simulink model "modelo_lqr_infinito"  (R2016a)
settings: Solver=VariableStepAuto  StartTime=0.0  StopTime=100  RelTol=1e-3
values from neighbouring files (symbols this model uses):
  A = [-0.1107 0; 0.1107 -0.1107]    [plantilla_lqr.m]
  B = [-1 1;0 0]    [plantilla_lqr.m]
undefined symbols (not defined in the file or in its folder): K
settings Model: Creator=Juan Pablo Requez  LastModifiedBy=Juan Pablo Requez

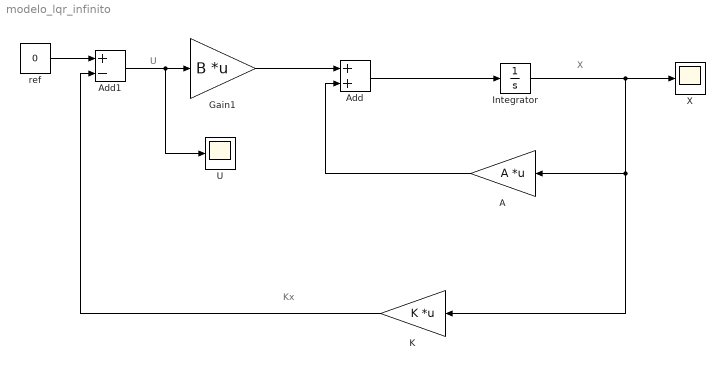
== system modelo_lqr_infinito ==
  note: Kx
  note: U
  note: X
  A : Gain  Gain=A  Multiplication=Matrix(K*u)
  Add : Sum
  Add1 : Sum  Inputs=+-
  Gain1 : Gain  Gain=B  Multiplication=Matrix(K*u)
  Integrator : Integrator  InitialCondition=[0.1 0.1]
  K : Gain  Gain=K  Multiplication=Matrix(K*u)
  U : Scope
  X : Scope
  ref : Constant  Value=0
  wires:
  Integrator/1 -> K/1, A/1, X/1
  A/1 -> Add/2
  Gain1/1 -> Add/1
  Add/1 -> Integrator/1
  Add1/1 -> U/1, Gain1/1
  ref/1 -> Add1/1
  K/1 -> Add1/2
